simulink model "generic_src"  (Simulink 10.1)
settings: Solver=ode45  StartTime=0.0  StopTime=inf  RelTol=1e-3  EnableMultiTasking=on
libraries: CarMaker4SL x4, simulink x3
(part 5 of 5)

== system generic_src/CarMaker/IPG Vehicle/PowerTrain/TCU Example/PTTransmCU_In/CreateBus TCU_Cfg GearBoxM0 ==
  In : Inport
  BusCreator : BusCreator  Inputs=38
  Demux : Demux  Outputs=38
      settings: DisplayOption=none
  Out : Outport  VectorParamsAs1DForOutWhenUnconnected=off
  wires:
  Demux/38 -> BusCreator/38  "TCU_Cfg GearBoxM0 iBGear16"
  Demux/37 -> BusCreator/37  "TCU_Cfg GearBoxM0 iBGear15"
  Demux/36 -> BusCreator/36  "TCU_Cfg GearBoxM0 iBGear14"
  Demux/35 -> BusCreator/35  "TCU_Cfg GearBoxM0 iBGear13"
  Demux/34 -> BusCreator/34  "TCU_Cfg GearBoxM0 iBGear12"
  Demux/33 -> BusCreator/33  "TCU_Cfg GearBoxM0 iBGear11"
  Demux/32 -> BusCreator/32  "TCU_Cfg GearBoxM0 iBGear10"
  Demux/31 -> BusCreator/31  "TCU_Cfg GearBoxM0 iBGear9"
  Demux/30 -> BusCreator/30  "TCU_Cfg GearBoxM0 iBGear8"
  Demux/29 -> BusCreator/29  "TCU_Cfg GearBoxM0 iBGear7"
  Demux/28 -> BusCreator/28  "TCU_Cfg GearBoxM0 iBGear6"
  Demux/27 -> BusCreator/27  "TCU_Cfg GearBoxM0 iBGear5"
  Demux/26 -> BusCreator/26  "TCU_Cfg GearBoxM0 iBGear4"
  Demux/25 -> BusCreator/25  "TCU_Cfg GearBoxM0 iBGear3"
  Demux/24 -> BusCreator/24  "TCU_Cfg GearBoxM0 iBGear2"
  Demux/23 -> BusCreator/23  "TCU_Cfg GearBoxM0 iBGear1"
  Demux/22 -> BusCreator/22  "TCU_Cfg GearBoxM0 iBGear0"
  Demux/21 -> BusCreator/21  "TCU_Cfg GearBoxM0 nBGears"
  Demux/20 -> BusCreator/20  "TCU_Cfg GearBoxM0 iFGear16"
  Demux/19 -> BusCreator/19  "TCU_Cfg GearBoxM0 iFGear15"
  Demux/18 -> BusCreator/18  "TCU_Cfg GearBoxM0 iFGear14"
  Demux/17 -> BusCreator/17  "TCU_Cfg GearBoxM0 iFGear13"
  Demux/16 -> BusCreator/16  "TCU_Cfg GearBoxM0 iFGear12"
  Demux/15 -> BusCreator/15  "TCU_Cfg GearBoxM0 iFGear11"
  Demux/14 -> BusCreator/14  "TCU_Cfg GearBoxM0 iFGear10"
  Demux/13 -> BusCreator/13  "TCU_Cfg GearBoxM0 iFGear9"
  Demux/12 -> BusCreator/12  "TCU_Cfg GearBoxM0 iFGear8"
  Demux/11 -> BusCreator/11  "TCU_Cfg GearBoxM0 iFGear7"
  Demux/10 -> BusCreator/10  "TCU_Cfg GearBoxM0 iFGear6"
  Demux/9 -> BusCreator/9  "TCU_Cfg GearBoxM0 iFGear5"
  Demux/8 -> BusCreator/8  "TCU_Cfg GearBoxM0 iFGear4"
  Demux/7 -> BusCreator/7  "TCU_Cfg GearBoxM0 iFGear3"
  Demux/6 -> BusCreator/6  "TCU_Cfg GearBoxM0 iFGear2"
  Demux/5 -> BusCreator/5  "TCU_Cfg GearBoxM0 iFGear1"
  Demux/4 -> BusCreator/4  "TCU_Cfg GearBoxM0 iFGear0"
  Demux/3 -> BusCreator/3  "TCU_Cfg GearBoxM0 nFGears"
  Demux/2 -> BusCreator/2  "TCU_Cfg GearBoxM0 ClKind"
  Demux/1 -> BusCreator/1  "TCU_Cfg GearBoxM0 GBKind"
  BusCreator/1 -> Out/1
  In/1 -> Demux/1

== system generic_src/CarMaker/IPG Vehicle/PowerTrain/TCU Example/PTTransmCU_In/CreateBus TCU_Cfg GearBoxM1 ==
  In : Inport
  BusCreator : BusCreator  Inputs=38
  Demux : Demux  Outputs=38
      settings: DisplayOption=none
  Out : Outport  VectorParamsAs1DForOutWhenUnconnected=off
  wires:
  Demux/38 -> BusCreator/38  "TCU_Cfg GearBoxM1 iBGear16"
  Demux/37 -> BusCreator/37  "TCU_Cfg GearBoxM1 iBGear15"
  Demux/36 -> BusCreator/36  "TCU_Cfg GearBoxM1 iBGear14"
  Demux/35 -> BusCreator/35  "TCU_Cfg GearBoxM1 iBGear13"
  Demux/34 -> BusCreator/34  "TCU_Cfg GearBoxM1 iBGear12"
  Demux/33 -> BusCreator/33  "TCU_Cfg GearBoxM1 iBGear11"
  Demux/32 -> BusCreator/32  "TCU_Cfg GearBoxM1 iBGear10"
  Demux/31 -> BusCreator/31  "TCU_Cfg GearBoxM1 iBGear9"
  Demux/30 -> BusCreator/30  "TCU_Cfg GearBoxM1 iBGear8"
  Demux/29 -> BusCreator/29  "TCU_Cfg GearBoxM1 iBGear7"
  Demux/28 -> BusCreator/28  "TCU_Cfg GearBoxM1 iBGear6"
  Demux/27 -> BusCreator/27  "TCU_Cfg GearBoxM1 iBGear5"
  Demux/26 -> BusCreator/26  "TCU_Cfg GearBoxM1 iBGear4"
  Demux/25 -> BusCreator/25  "TCU_Cfg GearBoxM1 iBGear3"
  Demux/24 -> BusCreator/24  "TCU_Cfg GearBoxM1 iBGear2"
  Demux/23 -> BusCreator/23  "TCU_Cfg GearBoxM1 iBGear1"
  Demux/22 -> BusCreator/22  "TCU_Cfg GearBoxM1 iBGear0"
  Demux/21 -> BusCreator/21  "TCU_Cfg GearBoxM1 nBGears"
  Demux/20 -> BusCreator/20  "TCU_Cfg GearBoxM1 iFGear16"
  Demux/19 -> BusCreator/19  "TCU_Cfg GearBoxM1 iFGear15"
  Demux/18 -> BusCreator/18  "TCU_Cfg GearBoxM1 iFGear14"
  Demux/17 -> BusCreator/17  "TCU_Cfg GearBoxM1 iFGear13"
  Demux/16 -> BusCreator/16  "TCU_Cfg GearBoxM1 iFGear12"
  Demux/15 -> BusCreator/15  "TCU_Cfg GearBoxM1 iFGear11"
  Demux/14 -> BusCreator/14  "TCU_Cfg GearBoxM1 iFGear10"
  Demux/13 -> BusCreator/13  "TCU_Cfg GearBoxM1 iFGear9"
  Demux/12 -> BusCreator/12  "TCU_Cfg GearBoxM1 iFGear8"
  Demux/11 -> BusCreator/11  "TCU_Cfg GearBoxM1 iFGear7"
  Demux/10 -> BusCreator/10  "TCU_Cfg GearBoxM1 iFGear6"
  Demux/9 -> BusCreator/9  "TCU_Cfg GearBoxM1 iFGear5"
  Demux/8 -> BusCreator/8  "TCU_Cfg GearBoxM1 iFGear4"
  Demux/7 -> BusCreator/7  "TCU_Cfg GearBoxM1 iFGear3"
  Demux/6 -> BusCreator/6  "TCU_Cfg GearBoxM1 iFGear2"
  Demux/5 -> BusCreator/5  "TCU_Cfg GearBoxM1 iFGear1"
  Demux/4 -> BusCreator/4  "TCU_Cfg GearBoxM1 iFGear0"
  Demux/3 -> BusCreator/3  "TCU_Cfg GearBoxM1 nFGears"
  Demux/2 -> BusCreator/2  "TCU_Cfg GearBoxM1 ClKind"
  Demux/1 -> BusCreator/1  "TCU_Cfg GearBoxM1 GBKind"
  BusCreator/1 -> Out/1
  In/1 -> Demux/1

== system generic_src/CarMaker/IPG Vehicle/PowerTrain/TCU Example/PTTransmCU_In/CreateBus TCU_Cfg GearBoxM2 ==
  In : Inport
  BusCreator : BusCreator  Inputs=38
  Demux : Demux  Outputs=38
      settings: DisplayOption=none
  Out : Outport  VectorParamsAs1DForOutWhenUnconnected=off
  wires:
  Demux/38 -> BusCreator/38  "TCU_Cfg GearBoxM2 iBGear16"
  Demux/37 -> BusCreator/37  "TCU_Cfg GearBoxM2 iBGear15"
  Demux/36 -> BusCreator/36  "TCU_Cfg GearBoxM2 iBGear14"
  Demux/35 -> BusCreator/35  "TCU_Cfg GearBoxM2 iBGear13"
  Demux/34 -> BusCreator/34  "TCU_Cfg GearBoxM2 iBGear12"
  Demux/33 -> BusCreator/33  "TCU_Cfg GearBoxM2 iBGear11"
  Demux/32 -> BusCreator/32  "TCU_Cfg GearBoxM2 iBGear10"
  Demux/31 -> BusCreator/31  "TCU_Cfg GearBoxM2 iBGear9"
  Demux/30 -> BusCreator/30  "TCU_Cfg GearBoxM2 iBGear8"
  Demux/29 -> BusCreator/29  "TCU_Cfg GearBoxM2 iBGear7"
  Demux/28 -> BusCreator/28  "TCU_Cfg GearBoxM2 iBGear6"
  Demux/27 -> BusCreator/27  "TCU_Cfg GearBoxM2 iBGear5"
  Demux/26 -> BusCreator/26  "TCU_Cfg GearBoxM2 iBGear4"
  Demux/25 -> BusCreator/25  "TCU_Cfg GearBoxM2 iBGear3"
  Demux/24 -> BusCreator/24  "TCU_Cfg GearBoxM2 iBGear2"
  Demux/23 -> BusCreator/23  "TCU_Cfg GearBoxM2 iBGear1"
  Demux/22 -> BusCreator/22  "TCU_Cfg GearBoxM2 iBGear0"
  Demux/21 -> BusCreator/21  "TCU_Cfg GearBoxM2 nBGears"
  Demux/20 -> BusCreator/20  "TCU_Cfg GearBoxM2 iFGear16"
  Demux/19 -> BusCreator/19  "TCU_Cfg GearBoxM2 iFGear15"
  Demux/18 -> BusCreator/18  "TCU_Cfg GearBoxM2 iFGear14"
  Demux/17 -> BusCreator/17  "TCU_Cfg GearBoxM2 iFGear13"
  Demux/16 -> BusCreator/16  "TCU_Cfg GearBoxM2 iFGear12"
  Demux/15 -> BusCreator/15  "TCU_Cfg GearBoxM2 iFGear11"
  Demux/14 -> BusCreator/14  "TCU_Cfg GearBoxM2 iFGear10"
  Demux/13 -> BusCreator/13  "TCU_Cfg GearBoxM2 iFGear9"
  Demux/12 -> BusCreator/12  "TCU_Cfg GearBoxM2 iFGear8"
  Demux/11 -> BusCreator/11  "TCU_Cfg GearBoxM2 iFGear7"
  Demux/10 -> BusCreator/10  "TCU_Cfg GearBoxM2 iFGear6"
  Demux/9 -> BusCreator/9  "TCU_Cfg GearBoxM2 iFGear5"
  Demux/8 -> BusCreator/8  "TCU_Cfg GearBoxM2 iFGear4"
  Demux/7 -> BusCreator/7  "TCU_Cfg GearBoxM2 iFGear3"
  Demux/6 -> BusCreator/6  "TCU_Cfg GearBoxM2 iFGear2"
  Demux/5 -> BusCreator/5  "TCU_Cfg GearBoxM2 iFGear1"
  Demux/4 -> BusCreator/4  "TCU_Cfg GearBoxM2 iFGear0"
  Demux/3 -> BusCreator/3  "TCU_Cfg GearBoxM2 nFGears"
  Demux/2 -> BusCreator/2  "TCU_Cfg GearBoxM2 ClKind"
  Demux/1 -> BusCreator/1  "TCU_Cfg GearBoxM2 GBKind"
  BusCreator/1 -> Out/1
  In/1 -> Demux/1

== system generic_src/CarMaker/IPG Vehicle/PowerTrain/TCU Example/PTTransmCU_In/CreateBus TCU_Cfg GearBoxM3 ==
  In : Inport
  BusCreator : BusCreator  Inputs=38
  Demux : Demux  Outputs=38
      settings: DisplayOption=none
  Out : Outport  VectorParamsAs1DForOutWhenUnconnected=off
  wires:
  Demux/38 -> BusCreator/38  "TCU_Cfg GearBoxM3 iBGear16"
  Demux/37 -> BusCreator/37  "TCU_Cfg GearBoxM3 iBGear15"
  Demux/36 -> BusCreator/36  "TCU_Cfg GearBoxM3 iBGear14"
  Demux/35 -> BusCreator/35  "TCU_Cfg GearBoxM3 iBGear13"
  Demux/34 -> BusCreator/34  "TCU_Cfg GearBoxM3 iBGear12"
  Demux/33 -> BusCreator/33  "TCU_Cfg GearBoxM3 iBGear11"
  Demux/32 -> BusCreator/32  "TCU_Cfg GearBoxM3 iBGear10"
  Demux/31 -> BusCreator/31  "TCU_Cfg GearBoxM3 iBGear9"
  Demux/30 -> BusCreator/30  "TCU_Cfg GearBoxM3 iBGear8"
  Demux/29 -> BusCreator/29  "TCU_Cfg GearBoxM3 iBGear7"
  Demux/28 -> BusCreator/28  "TCU_Cfg GearBoxM3 iBGear6"
  Demux/27 -> BusCreator/27  "TCU_Cfg GearBoxM3 iBGear5"
  Demux/26 -> BusCreator/26  "TCU_Cfg GearBoxM3 iBGear4"
  Demux/25 -> BusCreator/25  "TCU_Cfg GearBoxM3 iBGear3"
  Demux/24 -> BusCreator/24  "TCU_Cfg GearBoxM3 iBGear2"
  Demux/23 -> BusCreator/23  "TCU_Cfg GearBoxM3 iBGear1"
  Demux/22 -> BusCreator/22  "TCU_Cfg GearBoxM3 iBGear0"
  Demux/21 -> BusCreator/21  "TCU_Cfg GearBoxM3 nBGears"
  Demux/20 -> BusCreator/20  "TCU_Cfg GearBoxM3 iFGear16"
  Demux/19 -> BusCreator/19  "TCU_Cfg GearBoxM3 iFGear15"
  Demux/18 -> BusCreator/18  "TCU_Cfg GearBoxM3 iFGear14"
  Demux/17 -> BusCreator/17  "TCU_Cfg GearBoxM3 iFGear13"
  Demux/16 -> BusCreator/16  "TCU_Cfg GearBoxM3 iFGear12"
  Demux/15 -> BusCreator/15  "TCU_Cfg GearBoxM3 iFGear11"
  Demux/14 -> BusCreator/14  "TCU_Cfg GearBoxM3 iFGear10"
  Demux/13 -> BusCreator/13  "TCU_Cfg GearBoxM3 iFGear9"
  Demux/12 -> BusCreator/12  "TCU_Cfg GearBoxM3 iFGear8"
  Demux/11 -> BusCreator/11  "TCU_Cfg GearBoxM3 iFGear7"
  Demux/10 -> BusCreator/10  "TCU_Cfg GearBoxM3 iFGear6"
  Demux/9 -> BusCreator/9  "TCU_Cfg GearBoxM3 iFGear5"
  Demux/8 -> BusCreator/8  "TCU_Cfg GearBoxM3 iFGear4"
  Demux/7 -> BusCreator/7  "TCU_Cfg GearBoxM3 iFGear3"
  Demux/6 -> BusCreator/6  "TCU_Cfg GearBoxM3 iFGear2"
  Demux/5 -> BusCreator/5  "TCU_Cfg GearBoxM3 iFGear1"
  Demux/4 -> BusCreator/4  "TCU_Cfg GearBoxM3 iFGear0"
  Demux/3 -> BusCreator/3  "TCU_Cfg GearBoxM3 nFGears"
  Demux/2 -> BusCreator/2  "TCU_Cfg GearBoxM3 ClKind"
  Demux/1 -> BusCreator/1  "TCU_Cfg GearBoxM3 GBKind"
  BusCreator/1 -> Out/1
  In/1 -> Demux/1

== system generic_src/CarMaker/IPG Vehicle/PowerTrain/TCU Example/PTTransmCU_In/CreateBus TCU_Cfg Misc ==
  In : Inport
  BusCreator : BusCreator  Inputs=3
  Demux : Demux  Outputs=3
      settings: DisplayOption=none
  Out : Outport  VectorParamsAs1DForOutWhenUnconnected=off
  wires:
  Demux/2 -> BusCreator/2  "TCU_Cfg nGearBoxM"
  Demux/1 -> BusCreator/1  "TCU_Cfg ClKind"
  BusCreator/1 -> Out/1
  In/1 -> Demux/1
  Demux/3 -> BusCreator/3  "TCU_Cfg nClutchM"

== system generic_src/CarMaker/IPG Vehicle/PowerTrain/TCU Example/TCU Example/Calculate GearNoTrg ==
  GearNo : Inport
  rotvRef : Inport  Port=2
  SelectorCtrl : Inport  Port=3
  lastGearNoTrg : Inport  Port=4
  ShiftingTable : Inport  Port=5
  nFGears : Inport  Port=6
  Abs : Abs
  Backwards : Subsystem  TreatAsAtomicUnit=on
  Bias : Bias  Bias=-1
  Bias1 : Bias  Bias=-2
  Constant : Constant
  Driving : Subsystem  TreatAsAtomicUnit=on
  Gain : Gain  Gain=3
  Lower Limit : MultiPortSwitch  DataPortOrder=Zero-based contiguous  Inputs=1  zeroidx=on
  Merge : Merge  Inputs=3
  Switch : Switch  Criteria=u2 ~= 0
  Switch Case : SwitchCase  CaseConditions={1,-1}
  Upper Limit : MultiPortSwitch  DataPortOrder=Zero-based contiguous  Inputs=1  zeroidx=on
  else : Subsystem  TreatAsAtomicUnit=on
  rpm2radsec : Gain  Gain=0.104719755
  rpm2radsec1 : Gain  Gain=0.104719755
  GearNoTrg : Outport  VectorParamsAs1DForOutWhenUnconnected=off
  wires:
  Constant/1 -> Switch/3
  Switch/1 -> Abs/1
  lastGearNoTrg/1 -> Driving/6(GearNoTrg_last)
  nFGears/1 -> Driving/5(nFGears)
  rpm2radsec1/1 -> Driving/3(Lower Limit)
  rpm2radsec/1 -> Driving/2(Upper Limit)
  rotvRef/1 -> Driving/4(rotvRef)
  Abs/1 -> Gain/1
  Switch Case/3 -> else/Action
  Switch Case/2 -> Backwards/Action
  Merge/1 -> GearNoTrg/1
  else/1(GearNoTrg) -> Merge/3
  Backwards/1(GearNoTrg) -> Merge/2
  Driving/1(GearNoTrg) -> Merge/1
  Switch Case/1 -> Driving/Action
  SelectorCtrl/1 -> Switch Case/1
  Lower Limit/1 -> rpm2radsec1/1
  GearNo/1 -> Switch/1, Switch/2, Driving/1(GearNo)
  Bias1/1 -> Lower Limit/1
  Gain/1 -> Bias1/1, Bias/1
  ShiftingTable/1 -> Lower Limit/2, Upper Limit/2
  Bias/1 -> Upper Limit/1
  Upper Limit/1 -> rpm2radsec/1

== system generic_src/CarMaker/IPG Vehicle/PowerTrain/TCU Example/TCU Example/Limit GearNoTrg ==
  GearNoTrg : Inport
  nGears : Inport  Port=2
  Bus Selector : BusSelector  OutputSignals=TCU_Cfg GearBox nFGears,TCU_Cfg GearBox nBGears
  Gain : Gain  Gain=-1
  Saturation Dynamic : simulink/Discontinuities/Saturation Dynamic  OutMin=[]  OutMax=[]  OutDataTypeStr=Inherit: Same as second input  OutDataType=sfix(16)  OutScaling=2^-10  DoSatur=off
  GearNoTrg_limited : Outport  VectorParamsAs1DForOutWhenUnconnected=off
  wires:
  nGears/1 -> Bus Selector/1
  Saturation Dynamic/1 -> GearNoTrg_limited/1
  Gain/1 -> Saturation Dynamic/3
  Bus Selector/2 -> Gain/1  "<TCU_Cfg GearBox nBGears>"
  Bus Selector/1 -> Saturation Dynamic/1  "<TCU_Cfg GearBox nFGears>"
  GearNoTrg/1 -> Saturation Dynamic/2

== system generic_src/CarMaker/IPG Vehicle/PowerTrain/TCU Example/TCU Example/Retrun Zero ==
  Bus Creator : BusCreator  Inputs=2
  Constant : Constant  Value=0
  Constant1 : Constant  Value=0
  GearBoxOut : Outport  VectorParamsAs1DForOutWhenUnconnected=off
  wires:
  Bus Creator/1 -> GearBoxOut/1
  Constant1/1 -> Bus Creator/2  "TCU GearBoxIn set_ParkBrake"
  Constant/1 -> Bus Creator/1  "TCU GearBoxIn GearNoTrg"

== system generic_src/CarMaker/IPG Vehicle/PowerTrain/TCU Example/TCU Example/Calculate GearNoTrg/Backwards ==
  Action Port : ActionPort
  Constant : Constant  Value=-1
  GearNoTrg : Outport  InitialOutput=-1  VectorParamsAs1DForOutWhenUnconnected=off
  wires:
  Constant/1 -> GearNoTrg/1

== system generic_src/CarMaker/IPG Vehicle/PowerTrain/TCU Example/TCU Example/Calculate GearNoTrg/Driving ==
  GearNo : Inport
  Upper Limit : Inport  Port=2
  Lower Limit : Inport  Port=3
  rotvRef : Inport  Port=4
  nFGears : Inport  Port=5
  GearNoTrg_last : Inport  Port=6
  Action Port : ActionPort
  Bias : Bias  Bias=-1
  Bias1 : Bias  Bias=1
  Constant : Constant
  Constant1 : Constant
  Subsystem : Subsystem
  Subsystem1 : Subsystem
  Switch : Switch  Criteria=u2 ~= 0
  Switch1 : Switch  Criteria=u2 ~= 0
  Switch2 : Switch  Criteria=u2 ~= 0
  Switch3 : Switch  Criteria=u2 > Threshold
  GearNoTrg : Outport  InitialOutput=1  VectorParamsAs1DForOutWhenUnconnected=off
  wires:
  Constant1/1 -> Switch3/3
  GearNoTrg_last/1 -> Switch3/1, Switch3/2
  Switch3/1 -> Switch1/3
  Lower Limit/1 -> Subsystem1/3(Lower Limit)
  Subsystem1/1(Out1) -> Switch1/2
  nFGears/1 -> Subsystem/4(nFGears)
  Upper Limit/1 -> Subsystem/3(Upper Limit)
  Subsystem/1(Out1) -> Switch2/2
  Bias1/1 -> Switch2/1
  Bias/1 -> Switch1/1
  Switch1/1 -> Switch2/3
  Switch2/1 -> Switch/1
  rotvRef/1 -> Subsystem1/1(rotvRef), Subsystem/1(rotvRef)
  Switch/1 -> GearNoTrg/1
  Constant/1 -> Switch/3
  GearNo/1 -> Switch/2, Subsystem1/2(GearNo), Subsystem/2(GearNo), Bias1/1, Bias/1

== system generic_src/CarMaker/IPG Vehicle/PowerTrain/TCU Example/TCU Example/Calculate GearNoTrg/else ==
  Action Port : ActionPort
  Constant : Constant  Value=0
  GearNoTrg : Outport  InitialOutput=0  VectorParamsAs1DForOutWhenUnconnected=off
  wires:
  Constant/1 -> GearNoTrg/1

== system generic_src/CarMaker/IPG Vehicle/PowerTrain/TCU Example/TCU Example/Calculate GearNoTrg/Driving/Subsystem ==
  rotvRef : Inport
  GearNo : Inport  Port=2
  Upper Limit : Inport  Port=3
  nFGears : Inport  Port=4
  Logical Operator : Logic  AllPortsSameDT=off  OutDataTypeStr=boolean
  Relational Operator1 : RelationalOperator  OutDataTypeStr=boolean  RndMeth=Nearest
  Relational Operator2 : RelationalOperator  Operator=<  OutDataTypeStr=boolean  RndMeth=Nearest
  Out1 : Outport  VectorParamsAs1DForOutWhenUnconnected=off
  wires:
  Relational Operator2/1 -> Logical Operator/2
  nFGears/1 -> Relational Operator2/2
  GearNo/1 -> Relational Operator2/1
  Logical Operator/1 -> Out1/1
  Relational Operator1/1 -> Logical Operator/1
  Upper Limit/1 -> Relational Operator1/2
  rotvRef/1 -> Relational Operator1/1

== system generic_src/CarMaker/IPG Vehicle/PowerTrain/TCU Example/TCU Example/Calculate GearNoTrg/Driving/Subsystem1 ==
  rotvRef : Inport
  GearNo : Inport  Port=2
  Lower Limit : Inport  Port=3
  Constant : Constant
  Logical Operator : Logic  AllPortsSameDT=off  OutDataTypeStr=boolean
  Relational Operator1 : RelationalOperator  Operator=<=  OutDataTypeStr=boolean  RndMeth=Nearest
  Relational Operator2 : RelationalOperator  Operator=>  OutDataTypeStr=boolean  RndMeth=Nearest
  Out1 : Outport  VectorParamsAs1DForOutWhenUnconnected=off
  wires:
  Relational Operator2/1 -> Logical Operator/2
  Constant/1 -> Relational Operator2/2
  GearNo/1 -> Relational Operator2/1
  Logical Operator/1 -> Out1/1
  Relational Operator1/1 -> Logical Operator/1
  Lower Limit/1 -> Relational Operator1/2
  rotvRef/1 -> Relational Operator1/1
